simulink model "integrator_12B_with_contracts_Req_TUI003v3_SLDV_with_epsilon"  (R2019b)
settings: Solver=FixedStepDiscrete  StartTime=0.0  StopTime=10.0  FixedStep=1  RelTol=1e-3  EnableMultiTasking=on
model workspace (MAT data in the model file):
  ContractValidatorBlocksMap = containers.Map
  ContractValidatorBlocksMap.serialization.keys = {'integrator_12B/contract/validator', 'integrator_12B_with_contracts/integrator_12B_Tustin_IntegratorSpec/validator', 'integrator_12B_with_contracts_Req_TUI003v3/integrator_12B_Tustin_IntegratorSpec/validator'}
  ContractValidatorBlocksMap.serialization.values{1}.block = 'integrator_12B/contract/validator'
  ContractValidatorBlocksMap.serialization.values{1}.assumePorts = 0
  ContractValidatorBlocksMap.serialization.values{1}.guaranteePorts = 3
  ContractValidatorBlocksMap.serialization.values{1}.modeBlocksPorts = 0
  ContractValidatorBlocksMap.serialization.values{1}.portHandles.Inport = [741.001708984 742.001708984 743.001708984]
  ContractValidatorBlocksMap.serialization.values{1}.portHandles.Outport = 744.001708984
  ContractValidatorBlocksMap.serialization.values{1}.portHandles.Enable = []
  ContractValidatorBlocksMap.serialization.values{1}.portHandles.Trigger = []
  ContractValidatorBlocksMap.serialization.values{1}.portHandles.State = []
  ContractValidatorBlocksMap.serialization.values{1}.portHandles.LConn = []
  ContractValidatorBlocksMap.serialization.values{1}.portHandles.RConn = []
  ContractValidatorBlocksMap.serialization.values{1}.portHandles.Ifaction = []
  ContractValidatorBlocksMap.serialization.values{1}.portHandles.Reset = []
  ContractValidatorBlocksMap.serialization.values{1}.portConnectivity(1).Type = '1'
  ContractValidatorBlocksMap.serialization.values{1}.portConnectivity(1).Position = [365 -95]
  ContractValidatorBlocksMap.serialization.values{1}.portConnectivity(1).SrcBlock = 540.001953125
  ContractValidatorBlocksMap.serialization.values{1}.portConnectivity(1).SrcPort = 0
  ContractValidatorBlocksMap.serialization.values{1}.portConnectivity(1).DstBlock = []
  ContractValidatorBlocksMap.serialization.values{1}.portConnectivity(1).DstPort = []
  ContractValidatorBlocksMap.serialization.values{1}.portConnectivity(2).Type = '2'
  ContractValidatorBlocksMap.serialization.values{1}.portConnectivity(2).Position = [365 75]
  ContractValidatorBlocksMap.serialization.values{1}.portConnectivity(2).SrcBlock = 544.001953125
  ContractValidatorBlocksMap.serialization.values{1}.portConnectivity(2).SrcPort = 0
  ContractValidatorBlocksMap.serialization.values{1}.portConnectivity(2).DstBlock = []
  ContractValidatorBlocksMap.serialization.values{1}.portConnectivity(2).DstPort = []
  ContractValidatorBlocksMap.serialization.values{1}.portConnectivity(3).Type = '3'
  ContractValidatorBlocksMap.serialization.values{1}.portConnectivity(3).Position = [365 245]
  ContractValidatorBlocksMap.serialization.values{1}.portConnectivity(3).SrcBlock = 548.001953125
  ContractValidatorBlocksMap.serialization.values{1}.portConnectivity(3).SrcPort = 0
  ContractValidatorBlocksMap.serialization.values{1}.portConnectivity(3).DstBlock = []
  ContractValidatorBlocksMap.serialization.values{1}.portConnectivity(3).DstPort = []
  ContractValidatorBlocksMap.serialization.values{1}.portConnectivity(4).Type = '1'
  ContractValidatorBlocksMap.serialization.values{1}.portConnectivity(4).Position = [500 75]
  ContractValidatorBlocksMap.serialization.values{1}.portConnectivity(4).SrcBlock = []
  ContractValidatorBlocksMap.serialization.values{1}.portConnectivity(4).SrcPort = []
  ContractValidatorBlocksMap.serialization.values{1}.portConnectivity(4).DstBlock = 591.001708984
  ContractValidatorBlocksMap.serialization.values{1}.portConnectivity(4).DstPort = 0
  ContractValidatorBlocksMap.serialization.values{2}.block = 'integrator_12B_with_contracts/integrator_12B_Tustin_IntegratorSpec/validator'
  ContractValidatorBlocksMap.serialization.values{2}.assumePorts = 1
  ContractValidatorBlocksMap.serialization.values{2}.guaranteePorts = 1
  ContractValidatorBlocksMap.serialization.values{2}.modeBlocksPorts = 0
  ContractValidatorBlocksMap.serialization.values{2}.portHandles.Inport = [980.204833984 982.204833984]
  ContractValidatorBlocksMap.serialization.values{2}.portHandles.Outport = 1004.20471191
  ContractValidatorBlocksMap.serialization.values{2}.portHandles.Enable = []
  ContractValidatorBlocksMap.serialization.values{2}.portHandles.Trigger = []
  ContractValidatorBlocksMap.serialization.values{2}.portHandles.State = []
  ContractValidatorBlocksMap.serialization.values{2}.portHandles.LConn = []
  ContractValidatorBlocksMap.serialization.values{2}.portHandles.RConn = []
  ContractValidatorBlocksMap.serialization.values{2}.portHandles.Ifaction = []
  ContractValidatorBlocksMap.serialization.values{2}.portHandles.Reset = []
  ContractValidatorBlocksMap.serialization.values{2}.portConnectivity(1).Type = '1'
  ContractValidatorBlocksMap.serialization.values{2}.portConnectivity(1).Position = [1560 730]
  ContractValidatorBlocksMap.serialization.values{2}.portConnectivity(1).SrcBlock = 717.204711914
  ContractValidatorBlocksMap.serialization.values{2}.portConnectivity(1).SrcPort = 0
  ContractValidatorBlocksMap.serialization.values{2}.portConnectivity(1).DstBlock = []
  ContractValidatorBlocksMap.serialization.values{2}.portConnectivity(1).DstPort = []
  ContractValidatorBlocksMap.serialization.values{2}.portConnectivity(2).Type = '2'
  ContractValidatorBlocksMap.serialization.values{2}.portConnectivity(2).Position = [1560 780]
  ContractValidatorBlocksMap.serialization.values{2}.portConnectivity(2).SrcBlock = 724.204711914
  ContractValidatorBlocksMap.serialization.values{2}.portConnectivity(2).SrcPort = 0
  ContractValidatorBlocksMap.serialization.values{2}.portConnectivity(2).DstBlock = []
  ContractValidatorBlocksMap.serialization.values{2}.portConnectivity(2).DstPort = []
  ContractValidatorBlocksMap.serialization.values{2}.portConnectivity(3).Type = '1'
  ContractValidatorBlocksMap.serialization.values{2}.portConnectivity(3).Position = [1600 755]
  ContractValidatorBlocksMap.serialization.values{2}.portConnectivity(3).SrcBlock = []
  ContractValidatorBlocksMap.serialization.values{2}.portConnectivity(3).SrcPort = []
  ContractValidatorBlocksMap.serialization.values{2}.portConnectivity(3).DstBlock = 781.204711914
  ContractValidatorBlocksMap.serialization.values{2}.portConnectivity(3).DstPort = 0
  ContractValidatorBlocksMap.serialization.values{3}.block = 'integrator_12B_with_contracts_Req_TUI003v3/integrator_12B_Tustin_IntegratorSpec/validator'
  ContractValidatorBlocksMap.serialization.values{3}.assumePorts = 1
  ContractValidatorBlocksMap.serialization.values{3}.guaranteePorts = 1
  ContractValidatorBlocksMap.serialization.values{3}.modeBlocksPorts = 0
  ContractValidatorBlocksMap.serialization.values{3}.portHandles.Inport = [2423.00720215 2424.00720215]
  ContractValidatorBlocksMap.serialization.values{3}.portHandles.Outport = 2425.00720215
  ContractValidatorBlocksMap.serialization.values{3}.portHandles.Enable = []
  ContractValidatorBlocksMap.serialization.values{3}.portHandles.Trigger = []
  ContractValidatorBlocksMap.serialization.values{3}.portHandles.State = []
  ContractValidatorBlocksMap.serialization.values{3}.portHandles.LConn = []
  ContractValidatorBlocksMap.serialization.values{3}.portHandles.RConn = []
  ContractValidatorBlocksMap.serialization.values{3}.portHandles.Ifaction = []
  ContractValidatorBlocksMap.serialization.values{3}.portHandles.Reset = []
  ContractValidatorBlocksMap.serialization.values{3}.portConnectivity(1).Type = '1'
  ContractValidatorBlocksMap.serialization.values{3}.portConnectivity(1).Position = [1560 730]
  ContractValidatorBlocksMap.serialization.values{3}.portConnectivity(1).SrcBlock = 2174.00720215
  ContractValidatorBlocksMap.serialization.values{3}.portConnectivity(1).SrcPort = 0
  ContractValidatorBlocksMap.serialization.values{3}.portConnectivity(1).DstBlock = []
  ContractValidatorBlocksMap.serialization.values{3}.portConnectivity(1).DstPort = []
  ContractValidatorBlocksMap.serialization.values{3}.portConnectivity(2).Type = '2'
  ContractValidatorBlocksMap.serialization.values{3}.portConnectivity(2).Position = [1560 780]
  ContractValidatorBlocksMap.serialization.values{3}.portConnectivity(2).SrcBlock = 2168.00720215
  ContractValidatorBlocksMap.serialization.values{3}.portConnectivity(2).SrcPort = 0
  ContractValidatorBlocksMap.serialization.values{3}.portConnectivity(2).DstBlock = []
  ContractValidatorBlocksMap.serialization.values{3}.portConnectivity(2).DstPort = []
  ContractValidatorBlocksMap.serialization.values{3}.portConnectivity(3).Type = '1'
  ContractValidatorBlocksMap.serialization.values{3}.portConnectivity(3).Position = [1600 755]
  ContractValidatorBlocksMap.serialization.values{3}.portConnectivity(3).SrcBlock = []
  ContractValidatorBlocksMap.serialization.values{3}.portConnectivity(3).SrcPort = []
  ContractValidatorBlocksMap.serialization.values{3}.portConnectivity(3).DstBlock = 2196.00708008
  ContractValidatorBlocksMap.serialization.values{3}.portConnectivity(3).DstPort = 0
  ContractValidatorBlocksMap.serialization.uniformity = 0
  ContractValidatorBlocksMap.serialization.keyType = 'char'
  ContractValidatorBlocksMap.serialization.valueType = 'any'
libraries: sldvlib x2, simulink x1, cocosimLibs x1
settings Model: Creator=elliocm  LastModifiedBy=hbourbou
settings DataIOCC: LimitDataPoints=on  SaveFormat=Array  ReturnWorkspaceOutputs=off
settings OptimizationCC: ExpressionDepthLimit=2147483647  LifeSpan=inf
settings DebuggingCC: UnderspecifiedInitializationDetection=Classic  MergeDetectMultiDrivingBlocksExec=none  SolverPrmCheckMsg=warning  IntegerOverflowMsg=none  StateNameClashWarn=warning  SFUnexpectedBacktrackingDiag=warning  SFNoUnconditionalDefaultTransitionDiag=warning  SFExecutionAtInitializationDiag=none  IntegerSaturationMsg=none  ArithmeticOperatorsInVariantConditions=warning
settings HardwareCC: ProdBitPerPointer=32  ProdBitPerSizeT=32  ProdBitPerPtrDiffT=32  ProdLargestAtomicFloat=None  ProdIntDivRoundTo=Undefined  ProdEndianess=Unspecified  ProdWordSize=32  ProdHWDeviceType=32-bit Generic
settings ModelReferenceCC: PropagateSignalLabelsOutOfModel=off
settings SFSimCC: SimUseLocalCustomCode=off  CustomCodeUndefinedFunction=UseInterfaceOnly
settings RTWCC: RTWUseLocalCustomCode=off
settings CodeAppCC: StateflowObjectComments=on
settings GRTTargetCC: TargetLangStandard=C89/C90 (ANSI)  GeneratePreprocessorConditionals=Disable all
settings ConfigComp: CovMetricSettings=dw  CovHtmlReporting=on  CovSaveCumulativeToWorkspaceVar=on  CovSaveSingleToWorkspaceVar=on  CovExternalEMLEnable=off  DVMode=PropertyProving  DVMaxProcessTime=5000  DVMaxTestCaseSteps=500  DVTestSuiteOptimization=CombinedObjectives (Nonlinear Extended)  DVDetectActiveLogic=on

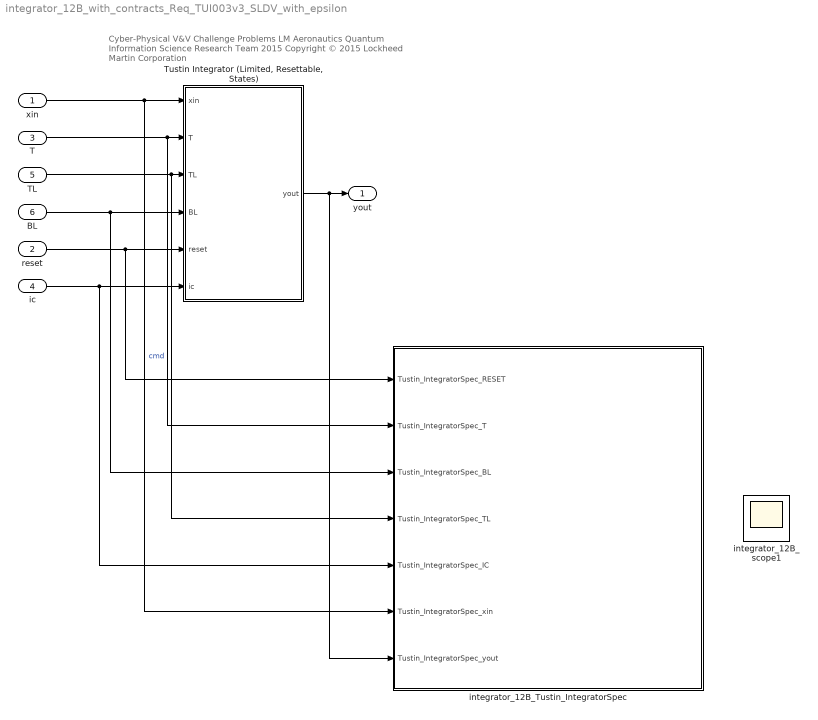
== system integrator_12B_with_contracts_Req_TUI003v3_SLDV_with_epsilon ==
  note: Cyber-Physical V&V Challenge Problems
      | LM Aeronautics Quantum Information Science Research Team 2015
      | Copyright © 2015 Lockheed Martin Corporation
  xin : Inport  OutDataTypeStr=double
  reset : Inport  Port=2  OutDataTypeStr=boolean
  T : Inport  Port=3  OutDataTypeStr=double
  ic : Inport  Port=4  OutDataTypeStr=double
  TL : Inport  Port=5  OutDataTypeStr=double
  BL : Inport  Port=6  OutDataTypeStr=double
  "Tustin Integrator (Limited, Resettable, States)" : Subsystem
  integrator_12B_Tustin_IntegratorSpec : Subsystem  TreatAsAtomicUnit=on  SimViewingDevice=on  mask(VerificationSubsystem){}
      mask Display: image(imread('sldvicon_versubsys.png','BackGroundColor',[1 1 1]),'center');
  integrator_12B_scope1 : Scope
  yout : Outport  VectorParamsAs1DForOutWhenUnconnected=off
  wires:
  BL/1 -> integrator_12B_Tustin_IntegratorSpec/3(Tustin_IntegratorSpec_BL), "Tustin Integrator (Limited, Resettable, States)"/4(BL)
  TL/1 -> "Tustin Integrator (Limited, Resettable, States)"/3(TL), integrator_12B_Tustin_IntegratorSpec/4(Tustin_IntegratorSpec_TL)
  reset/1 -> integrator_12B_Tustin_IntegratorSpec/1(Tustin_IntegratorSpec_RESET), "Tustin Integrator (Limited, Resettable, States)"/5(reset)
  ic/1 -> integrator_12B_Tustin_IntegratorSpec/5(Tustin_IntegratorSpec_IC), "Tustin Integrator (Limited, Resettable, States)"/6(ic)
  "Tustin Integrator (Limited, Resettable, States)"/1(yout) -> yout/1, integrator_12B_Tustin_IntegratorSpec/7(Tustin_IntegratorSpec_yout)
  T/1 -> "Tustin Integrator (Limited, Resettable, States)"/2(T), integrator_12B_Tustin_IntegratorSpec/2(Tustin_IntegratorSpec_T)
  xin/1 -> "Tustin Integrator (Limited, Resettable, States)"/1(xin), integrator_12B_Tustin_IntegratorSpec/6(Tustin_IntegratorSpec_xin)  "cmd"
  ? -> integrator_12B_scope1/1

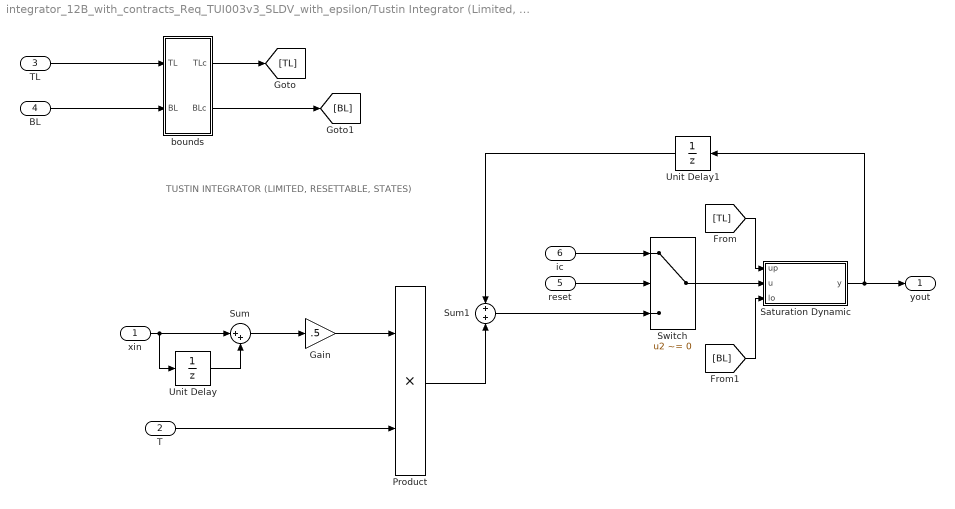
== system integrator_12B_with_contracts_Req_TUI003v3_SLDV_with_epsilon/Tustin Integrator (Limited, Resettable, States) ==
  note: TUSTIN INTEGRATOR (LIMITED, RESETTABLE, STATES)
  xin : Inport
  T : Inport  Port=2
  TL : Inport  Port=3
  BL : Inport  Port=4
  reset : Inport  Port=5
  ic : Inport  Port=6
  Gain : Gain  Gain=.5
  Product : Product  RndMeth=Zero
  Saturation Dynamic : Subsystem  mask(Saturation Dynamic){OutMin=[], OutMax=[], OutDataTypeStr=Inherit: Same as second input, OutputDataTypeScalingMode=Same as second input, OutDataType=fixdt(1, 16), OutScaling=2^-10, LockScale=off, RndMeth=Floor, DoSatur=off}
      mask prompts: OutMin "Simulink:masks:OutputMinimum_MP"; OutMax "Simulink:masks:OutputMaximum_MP"; OutDataTypeStr "Simulink:masks:OutputDataType_MP"; OutputDataTypeScalingMode "Simulink:masks:OutputDataTypeMode_MP"; OutDataType "Simulink:masks:OutputDataTypeegFixdt116Fixdtsingle_MP"; OutScaling "Simulink:masks:OutputScalingSlopeEg29OrSlopeBias_MP"; LockScale "Simulink:masks:LockOutputDataTypeAgainstFxpTools_MP"; RndMeth "Simulink:masks:IntegerRoundingMode_MP"; DoSatur "Simulink:masks:SaturateOnIntegerOverflow_MP"
      mask help: Simulink:masks:SaturationDynamic_MD
      mask init:
      | blkH = gcbh;
      | blkName = getfullname(blkH);
      | 
      | switch_blks = {'Switch','Switch2'}; 
      | for i = 1:length(switch_blks)
      |   set_param([blkName,'/',switch_blks{i}], ...
      |       'RndMeth', RndMeth, ...
      | 	  'DoSatur', DoSatur);
      | end
      | 
      | propBlk = [blkName, '/Data Type Propagation'];
      | 
      | if strcmp(OutputDataTypeScalingMode, 'Same as second input')
      |     set_param(propBlk, 'PropDataTypeMode', 'Inherit via propagation rule', ...
      |                        'PropScalingMode',  'Inherit via propagation rule');
      | else
      |     scaling = OutScaling;
      |     scalingMode = 'Specify via dialog';
      |     switch OutputDataTypeScalingMode
      |       case 'double'
      |         dataType = 'fixdt(''double'')';
      |       case 'single'
      |         dataType = 'fixdt(''single'')';
      |       case 'int8'
      |         dataType = 'fixdt(1,8,0)';
      |       case 'uint8'
      |         dataType = 'fixdt(0,8,0)';
      |       case 'int16'
      |         dataType = 'fixdt(1,16,0)';
      |       case 'uint16'
      |         dataType = 'fixdt(0,16,0)';
      |       case 'int32'
      |         dataType = 'fixdt(1,32,0)';
      |       case 'uint32'
      |         dataType = 'fixdt(0,32,0)';
      |       case 'Specify via dialog'
      |         dataType = OutDataType;
      |         if ~isempty(OutDataTypeStr) && isa(OutDataTypeStr,'Simulink.NumericType') 
      |           if strcmp(OutDataTypeStr.DataTypeMode, 'Fixed-point: unspecified scaling') 
      |             scalingMode = 'Obtain via best precision';
      |             range = [OutMin OutMax];
      |             range = range(~isinf(range));
      |             set_param(propBlk, 'ValuesUsedBestPrec', mat2str(range));
      |           end
      |         end
      |     end
      |     
      |     set_param(propBlk, 'PropDataTypeMode', 'Specify via dialog', ...
      |                        'PropScalingMode',  scalingMode, ...
      |                        'PropDataType',     dataType, ...
      |                        'PropScaling',      scaling);
      | end
      mask Callback OutDataTypeStr: fixptdialog(gcbh)
      mask TypeOptions OutputDataTypeScalingMode: double | single | int8 | uint8 | int16 | uint16 | int32 | uint32 | Specify via dialog | Same as second input
      mask Callback OutputDataTypeScalingMode: fixptdialog(gcbh)
      mask Callback OutDataType: fixptdialog(gcbh)
      mask TypeOptions RndMeth: Simulink:masks:Ceiling | Simulink:masks:Convergent | Simulink:masks:Floor | Simulink:masks:Nearest | Simulink:masks:Round | Simulink:masks:Simplest | Simulink:masks:Zero
  Sum : Sum  Inputs=|++
  Sum1 : Sum
  Switch : Switch  Criteria=u2 ~= 0  Threshold=0.5
  Unit Delay : UnitDelay  SampleTime=-1  HasFrameUpgradeWarning=on
  Unit Delay1 : UnitDelay  SampleTime=-1  HasFrameUpgradeWarning=on
  bounds : Subsystem
  yout : Outport  VectorParamsAs1DForOutWhenUnconnected=off
  wires:
  xin/1 -> Unit Delay/1, Sum/1
  Unit Delay/1 -> Sum/2
  Sum/1 -> Gain/1
  Gain/1 -> Product/1
  T/1 -> Product/2
  Product/1 -> Sum1/2
  Sum1/1 -> Switch/3
  reset/1 -> Switch/2
  ic/1 -> Switch/1
  Switch/1 -> Saturation Dynamic/2(u)
  Saturation Dynamic/1(y) -> Unit Delay1/1, yout/1
  Unit Delay1/1 -> Sum1/1
  TL/1 -> bounds/1(TL)
  BL/1 -> bounds/2(BL)
  bounds/1(TLc) -> [TL]
  bounds/2(BLc) -> [BL]
  [TL] -> Saturation Dynamic/1(up)
  [BL] -> Saturation Dynamic/3(lo)

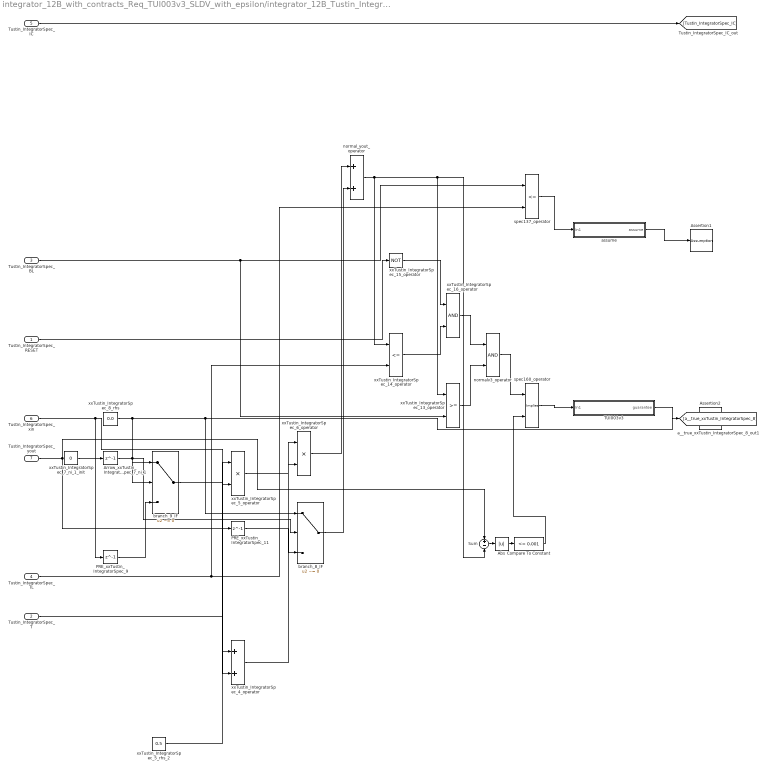
== system integrator_12B_with_contracts_Req_TUI003v3_SLDV_with_epsilon/integrator_12B_Tustin_IntegratorSpec ==
  Tustin_IntegratorSpec_RESET : Inport  OutDataTypeStr=boolean
  Tustin_IntegratorSpec_T : Inport  Port=2  OutDataTypeStr=double
  Tustin_IntegratorSpec_BL : Inport  Port=3  OutDataTypeStr=double
  Tustin_IntegratorSpec_TL : Inport  Port=4  OutDataTypeStr=double
  Tustin_IntegratorSpec_IC : Inport  Port=5  OutDataTypeStr=double
  Tustin_IntegratorSpec_xin : Inport  Port=6  OutDataTypeStr=double
  Tustin_IntegratorSpec_yout : Inport  Port=7  OutDataTypeStr=double
  Abs : Abs
  Arrow_xxTustin_IntegratorSpec_7_ni_1 : Delay  DelayLength=1  InitialCondition=1
  Assertion1 : sldvlib/Objectives and Constraints/Assumption  enabled=on  customAVTBlockType=Assumption  intervals=true  initial=off  dispValues=on  outEnabled=off
      settings: AttributesFormatString=%<intervals>  SourceProductName=Simulink  SourceProductBaseCode=SL
  Assertion2 : sldvlib/Objectives and Constraints/Proof Objective  enabled=on  customAVTBlockType=Proof Objective  intervals=true  dispValues=on  outEnabled=off  enableStopSim=off
      settings: AttributesFormatString=%<intervals>  SourceProductName=Simulink  SourceProductBaseCode=SL
  Compare To Constant : simulink/Logic and Bit Operations/Compare To Constant  relop=<=  const=0.001  OutDataTypeStr=boolean
  PRE_xxTustin_IntegratorSpec_11 : Delay  DelayLength=1  InitialCondition=0
  PRE_xxTustin_IntegratorSpec_9 : Delay  DelayLength=1  InitialCondition=0
  Sum : Sum  Inputs=+-
  TUI003v3 : Subsystem
  assume : Subsystem
  branch_8_IF : Switch  Criteria=u2 ~= 0
  branch_9_IF : Switch  Criteria=u2 ~= 0
  normal_yout_operator : Sum  OutDataTypeStr=double
  normalv3_operator : Logic  AllPortsSameDT=off  OutDataTypeStr=boolean
  spec137_operator : RelationalOperator  Operator=<=  OutDataTypeStr=boolean  RndMeth=Simplest
  spec160_operator : cocosimLibs/Implies  SystemSampleTime=-1  Latency=0  AutoFrameSizeCalculation=off
  xxTustin_IntegratorSpec_13_operator : RelationalOperator  OutDataTypeStr=boolean  RndMeth=Simplest
  xxTustin_IntegratorSpec_14_operator : RelationalOperator  Operator=<=  OutDataTypeStr=boolean  RndMeth=Simplest
  xxTustin_IntegratorSpec_15_operator : Logic  Operator=NOT  AllPortsSameDT=off  OutDataTypeStr=boolean
  xxTustin_IntegratorSpec_16_operator : Logic  AllPortsSameDT=off  OutDataTypeStr=boolean
  xxTustin_IntegratorSpec_4_operator : Sum  OutDataTypeStr=double
  xxTustin_IntegratorSpec_5_operator : Product  OutDataTypeStr=double
  xxTustin_IntegratorSpec_5_rhs_2 : Constant  Value=0.5  OutDataTypeStr=double
  xxTustin_IntegratorSpec_6_operator : Product  OutDataTypeStr=double
  xxTustin_IntegratorSpec_7_ni_1_init : Constant  Value=0  OutDataTypeStr=boolean
  xxTustin_IntegratorSpec_8_rhs : Constant  Value=0.0  OutDataTypeStr=double
  wires:
  xxTustin_IntegratorSpec_4_operator/1 -> xxTustin_IntegratorSpec_6_operator/2
  xxTustin_IntegratorSpec_5_operator/1 -> xxTustin_IntegratorSpec_6_operator/1
  xxTustin_IntegratorSpec_5_rhs_2/1 -> xxTustin_IntegratorSpec_5_operator/2
  Tustin_IntegratorSpec_T/1 -> xxTustin_IntegratorSpec_5_operator/1
  branch_9_IF/1 -> xxTustin_IntegratorSpec_4_operator/2
  xxTustin_IntegratorSpec_14_operator/1 -> xxTustin_IntegratorSpec_16_operator/2
  xxTustin_IntegratorSpec_15_operator/1 -> xxTustin_IntegratorSpec_16_operator/1
  Tustin_IntegratorSpec_RESET/1 -> xxTustin_IntegratorSpec_15_operator/1
  Compare To Constant/1 -> spec160_operator/2
  normalv3_operator/1 -> spec160_operator/1
  xxTustin_IntegratorSpec_13_operator/1 -> normalv3_operator/2
  xxTustin_IntegratorSpec_16_operator/1 -> normalv3_operator/1
  branch_8_IF/1 -> normal_yout_operator/2
  xxTustin_IntegratorSpec_6_operator/1 -> normal_yout_operator/1
  spec160_operator/1 -> TUI003v3/1(In1)
  PRE_xxTustin_IntegratorSpec_9/1 -> branch_9_IF/3
  PRE_xxTustin_IntegratorSpec_11/1 -> branch_8_IF/3
  spec137_operator/1 -> assume/1(In1)
  Tustin_IntegratorSpec_IC/1 -> [Tustin_IntegratorSpec_IC]
  xxTustin_IntegratorSpec_7_ni_1_init/1 -> Arrow_xxTustin_IntegratorSpec_7_ni_1/1
  Tustin_IntegratorSpec_yout/1 -> Sum/1, PRE_xxTustin_IntegratorSpec_11/1
  Tustin_IntegratorSpec_TL/1 -> xxTustin_IntegratorSpec_14_operator/2, spec137_operator/2
  Tustin_IntegratorSpec_BL/1 -> xxTustin_IntegratorSpec_13_operator/2, spec137_operator/1
  normal_yout_operator/1 -> Sum/2, xxTustin_IntegratorSpec_13_operator/1, xxTustin_IntegratorSpec_14_operator/1
  Tustin_IntegratorSpec_xin/1 -> xxTustin_IntegratorSpec_4_operator/1, PRE_xxTustin_IntegratorSpec_9/1
  xxTustin_IntegratorSpec_8_rhs/1 -> branch_8_IF/1, [a__true_xxTustin_IntegratorSpec_8], branch_9_IF/1
  Arrow_xxTustin_IntegratorSpec_7_ni_1/1 -> branch_9_IF/2, branch_8_IF/2
  assume/1(assume) -> Assertion1/1
  TUI003v3/1(guarantee) -> Assertion2/1
  Sum/1 -> Abs/1
  Abs/1 -> Compare To Constant/1

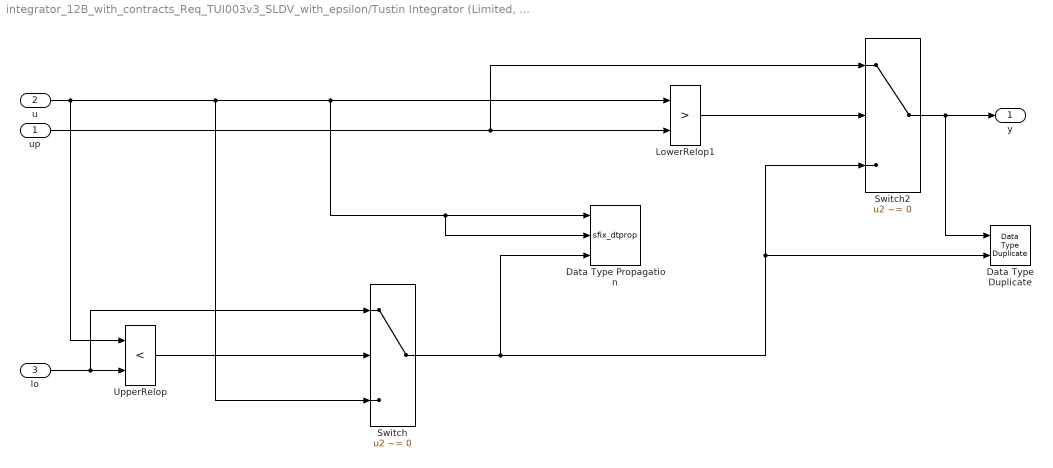
== system integrator_12B_with_contracts_Req_TUI003v3_SLDV_with_epsilon/Tustin Integrator (Limited, Resettable, States)/Saturation Dynamic ==
  up : Inport
  u : Inport  Port=2
  lo : Inport  Port=3
  Data Type Duplicate : DataTypeDuplicate  DisableCoverage=on
  Data Type Propagation : S-Function  FunctionName=sfix_dtprop  Parameters=14,PropDataTypeMode,(getdatatypespecs(PropDataType,PropScaling,DblOver,0, 0, PropDataTypeMode, PropScalingMode)),IfRefDouble,IfRefSingle,IsSigned,NumBitsBase,NumBitsMult,NumBitsAdd,(sort(reshape(round(NumBitsAllowFinal), prod(size(NumBitsAllowFinal)),1))),PropScalingMode,ValuesUsedBestPrec,SlopeBase,SlopeMult,SlopeAdd,BiasBase,BiasMult,BiasAdd,DblOver  SFunctionDeploymentMode=off  EnableBusSupport=off  mask(Data Type Propagation){PropDataTypeMode=Inherit via propagation rule, PropDataType=fixdt(1, 16), IfRefDouble=double, IfRefSingle=single, IsSigned=IsSigned1, NumBitsBase=NumBits1, NumBitsMult=1, NumBitsAdd=0, NumBitsAllowFinal=1:128, PropScalingMode=Inherit via propagation rule, PropScaling=2^-10, ValuesUsedBestPrec=[5 -7], SlopeBase=Slope1, SlopeMult=1, SlopeAdd=0, BiasBase=Bias1, BiasMult=1, BiasAdd=0}
      mask prompts: PropDataTypeMode "Simulink:masks:x1PropagatedDataType_MP"; PropDataType "Simulink:masks:x11PropagatedDataTypeegFixdt116Fixdtsingle_MP"; IfRefDouble "Simulink:masks:x11IfAnyReferenceInputIsDoubleOutputIs_MP"; IfRefSingle "Simulink:masks:x12IfAnyReferenceInputIsSingleOutputIs_MP"; IsSigned "Simulink:masks:x13IsSigned_MP"; NumBitsBase "Simulink:masks:x141NumberofBitsBase_MP"; NumBitsMult "Simulink:masks:x142NumberofBitsMultiplicativeAdjustment_MP"; NumBitsAdd "Simulink:masks:x143NumberofBitsAdditiveAdjustment_MP"; NumBitsAllowFinal "Simulink:masks:x144NumberofBitsAllowableFinalValues_MP"; PropScalingMode "Simulink:masks:x2PropagatedScaling_MP"; PropScaling "Simulink:masks:x21PropagatedScalingSlopeEg29OrSlopeBiasEg1253_MP"; ValuesUsedBestPrec "Simulink:masks:x21ValuesUsedToDetermineBestPrecisionScaling_MP"; SlopeBase "Simulink:masks:x211SlopeBase_MP"; SlopeMult "Simulink:masks:x212SlopeMultiplicativeAdjustment_MP"; SlopeAdd "Simulink:masks:x213SlopeAdditiveAdjustment_MP"; BiasBase "Simulink:masks:x221BiasBase_MP"; BiasMult "Simulink:masks:x222BiasMultiplicativeAdjustment_MP"; BiasAdd "Simulink:masks:x223BiasAdditiveAdjustment_MP"
      mask help: Simulink:masks:DataTypePropagation_MD
      mask init:
      | DblOver = 0;
      mask TypeOptions PropDataTypeMode: Simulink:masks:SpecifyViaDialog | Simulink:masks:InheritViaPropagationRule
      mask Callback PropDataTypeMode: fixptdialog(gcbh)
      mask Callback PropDataType: fixptdialog(gcbh)
      mask TypeOptions IfRefDouble: Simulink:masks:double | Simulink:masks:single
      mask TypeOptions IfRefSingle: Simulink:masks:double | Simulink:masks:single
      mask TypeOptions IsSigned: Simulink:masks:IsSigned1 | Simulink:masks:IsSigned2 | Simulink:masks:IsSigned1OrIsSigned2 | Simulink:masks:TRUE | Simulink:masks:FALSE
      mask TypeOptions NumBitsBase: NumBits1 | NumBits2 | max([NumBits1 NumBits2]) | min([NumBits1 NumBits2]) | NumBits1+NumBits2
      mask TypeOptions PropScalingMode: Simulink:masks:SpecifyViaDialog | Simulink:masks:InheritViaPropagationRule | Simulink:masks:ObtainViaBestPrecision
      mask Callback PropScalingMode: fixptdialog(gcbh)
      mask TypeOptions SlopeBase: Slope1 | Slope2 | max([Slope1 Slope2]) | min([Slope1 Slope2]) | Slope1*Slope2 | Slope1/Slope2 | PosRange1 | PosRange2 | max([PosRange1 PosRange2]) | min([PosRange1 PosRange2]) | PosRange1*PosRange2 | PosRange1/PosRange2
      mask TypeOptions BiasBase: Bias1 | Bias2 | max([Bias1 Bias2]) | min([Bias1 Bias2]) | Bias1*Bias2 | Bias1/Bias2 | Bias1+Bias2 | Bias1-Bias2
      mask Display:
      | port_label('Input',1,'Ref1');
      | port_label('Input',2,'Ref2');
      | port_label('Input',3,'Prop');
  LowerRelop1 : RelationalOperator  DisableCoverage=on  Operator=>  OutDataTypeStr=boolean  RndMeth=Nearest
  Switch : Switch  Criteria=u2 ~= 0  OutDataTypeStr=Inherit: Inherit via back propagation  ZeroCross=off
  Switch2 : Switch  Criteria=u2 ~= 0  OutMin=OutMin  OutMax=OutMax  OutDataTypeStr=Inherit: Inherit via back propagation  ZeroCross=off
  UpperRelop : RelationalOperator  DisableCoverage=on  Operator=<  OutDataTypeStr=boolean  RndMeth=Nearest
  y : Outport  OutMin=OutMin  OutMax=OutMax  VectorParamsAs1DForOutWhenUnconnected=off
  wires:
  up/1 -> Switch2/1, LowerRelop1/2
  u/1 -> Data Type Propagation/2, Data Type Propagation/1, LowerRelop1/1, Switch/3, UpperRelop/1
  lo/1 -> Switch/1, UpperRelop/2
  Switch/1 -> Data Type Duplicate/2, Switch2/3, Data Type Propagation/3
  Switch2/1 -> Data Type Duplicate/1, y/1
  LowerRelop1/1 -> Switch2/2
  UpperRelop/1 -> Switch/2

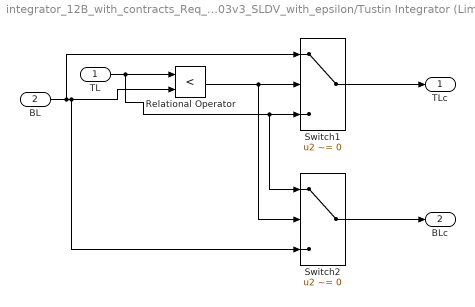
== system integrator_12B_with_contracts_Req_TUI003v3_SLDV_with_epsilon/Tustin Integrator (Limited, Resettable, States)/bounds ==
  TL : Inport
  BL : Inport  Port=2
  Relational Operator : RelationalOperator  Operator=<  OutDataTypeStr=boolean  RndMeth=Nearest
  Switch1 : Switch  Criteria=u2 ~= 0  Threshold=0.5
  Switch2 : Switch  Criteria=u2 ~= 0  Threshold=0.5
  TLc : Outport  VectorParamsAs1DForOutWhenUnconnected=off
  BLc : Outport  Port=2  VectorParamsAs1DForOutWhenUnconnected=off
  wires:
  BL/1 -> Switch1/1, Switch2/3, Relational Operator/2
  TL/1 -> Switch2/1, Switch1/3, Relational Operator/1
  Relational Operator/1 -> Switch2/2, Switch1/2
  Switch1/1 -> TLc/1
  Switch2/1 -> BLc/1

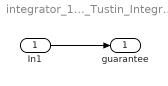
== system integrator_12B_with_contracts_Req_TUI003v3_SLDV_with_epsilon/integrator_12B_Tustin_IntegratorSpec/TUI003v3 ==
  In1 : Inport
  guarantee : Outport  OutDataTypeStr=boolean
  wires:
  In1/1 -> guarantee/1

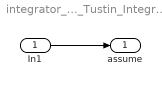
== system integrator_12B_with_contracts_Req_TUI003v3_SLDV_with_epsilon/integrator_12B_Tustin_IntegratorSpec/assume ==
  In1 : Inport
  assume : Outport  OutDataTypeStr=boolean
  wires:
  In1/1 -> assume/1
